simulink model "feedback_control"  (R2020b)
settings: Solver=FixedStepDiscrete  StartTime=0.0  StopTime=inf  FixedStep=step_size  RelTol=1e-3  EnableMultiTasking=on
libraries: arduinolib x1, dspstat3 x1, arduinosensorlib x1
settings Model: DataDictionary=data2.sldd  EnableAccessToBaseWorkspace=off  ModifiedByFormat=The MathWorks Inc.  SILPILModeSetting=veronly  ExtModeTrigDuration=2  Creator=The MathWorks, Inc.  LastModifiedBy=The MathWorks Inc.
settings DataIOCC: SaveFormat=Array  ReturnWorkspaceOutputs=off
settings OptimizationCC: PassReuseOutputArgsAs=Individual arguments  ExpressionDepthLimit=2147483647  ZeroExternalMemoryAtStartup=off  ZeroInternalMemoryAtStartup=off  EfficientFloat2IntCast=on  LifeSpan=1  MaxStackSize=64  EfficientTunableParamExpr=on
settings DebuggingCC: SolverPrmCheckMsg=warning  FcnCallInpInsideContextMsg=warning  UniqueDataStoreMsg=error  AssertControl=DisableAll  AllowSymbolicDim=off  StateNameClashWarn=warning  StrictBusMsg=ErrorOnBusTreatedAsVector  SFUnexpectedBacktrackingDiag=warning  SFNoUnconditionalDefaultTransitionDiag=warning  SFExecutionAtInitializationDiag=none  ArithmeticOperatorsInVariantConditions=warning
settings HardwareCC: ProdBitPerInt=16  ProdBitPerPointer=16  ProdBitPerSizeT=16  ProdBitPerPtrDiffT=16  ProdLargestAtomicFloat=None  ProdWordSize=8  ProdHWDeviceType=Atmel->AVR
settings ModelReferenceCC: PropagateSignalLabelsOutOfModel=off
settings SFSimCC: SimUseLocalCustomCode=off  CustomCodeUndefinedFunction=UseInterfaceOnly
settings RTWCC: Description=Embedded Coder  SystemTargetFile=ert.tlc  HardwareBoard=Arduino Uno  TemplateMakefile=ert_default_tmf  RTWUseLocalCustomCode=off  Toolchain=Arduino AVR  BuildConfiguration=Faster Runs  IncludeHyperlinkInReport=on  GenerateCodeMetricsReport=on
settings CodeAppCC: IgnoreCustomStorageClasses=off  IgnoreTestpoints=on  CustomSymbolStrType=$N$R$M  StateflowObjectComments=on  InternalIdentifier=Classic
settings ERTTargetCC: MultiwordLength=2048  SupportNonFinite=off  SupportContinuousTime=on  SupportVariableSizeSignals=on  ParenthesesLevel=Maximum  ExtModeStaticAllocSize=250  ConvertIfToSwitch=off  SuppressUnreachableDefaultCases=off
settings ConfigComp: CovMetricSettings=dw  CovSaveCumulativeToWorkspaceVar=on  CovSaveSingleToWorkspaceVar=on  CovExternalEMLEnable=off  CovSFcnEnable=off

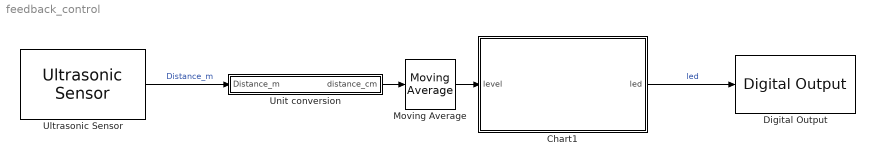
== system feedback_control ==
  Chart1 : Stateflow chart  TreatAsAtomicUnit=on
  Digital Output : arduinolib/Digital Output  pinNumber=13  Direction=output  blockPlatform=arduino
  Moving Average : dspstat3/Moving Average  Method=Sliding window  ForgettingFactorPort=off  SpecifyWindowLength=on  WindowLength=4  ForgettingFactor=0.9  SimulateUsing=Code generation
  Ultrasonic Sensor : arduinosensorlib/Ultrasonic Sensor  NumSignalPins=2  TrigPin=4  EchoPin=5  SignalPin=3  SampleTime_=0.1  blockPlatform=ARDUINO
      settings: SourceProductBaseCode=ARDUINO
  Unit conversion : Subsystem
  wires:
  Chart1/1(led) -> Digital Output/1  "led"
  Ultrasonic Sensor/1 -> Unit conversion/1(Distance_m)  "Distance_m"
  Unit conversion/1(distance_cm) -> Moving Average/1
  Moving Average/1 -> Chart1/1(level)

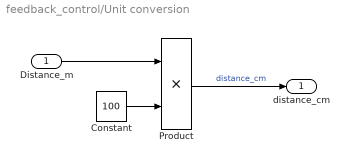
== system feedback_control/Unit conversion ==
  Distance_m : Inport
  Constant : Constant  Value=100
  Product : Product
  distance_cm : Outport
  wires:
  Product/1 -> distance_cm/1  "distance_cm"
  Distance_m/1 -> Product/1
  Constant/1 -> Product/2

== stateflow chart feedback_control/Chart1 ==
  state BLINK_OUTRANGE
    frequency = 0.5;
    state LED_OFF
      entry:
      led = false;
    state LED_ON
      entry:
      led = true;
    (default) -> BLINK_OUTRANGE.LED_ON
    BLINK_OUTRANGE.LED_ON -> BLINK_OUTRANGE.LED_OFF : after(frequency/2, sec)
    BLINK_OUTRANGE.LED_OFF -> BLINK_OUTRANGE.LED_ON : after(frequency/2, sec)
  state BLINK_INRANGE
    frequency = 0.1;
    state LED_OFF
      entry:
      led = false;
    state LED_ON
      entry:
      led = true;
    (default) -> BLINK_INRANGE.LED_ON
    BLINK_INRANGE.LED_OFF -> BLINK_INRANGE.LED_ON : after(frequency - ((level*frequency)/100), sec)
    BLINK_INRANGE.LED_ON -> BLINK_INRANGE.LED_OFF : after((level*frequency)/100, sec)
  state DISCONNECTED_SENSOR
    frequency = 1;
    state LED_OFF
      entry:
      led = false;
    state LED_ON
      entry:
      led = true;
    (default) -> DISCONNECTED_SENSOR.LED_ON
    DISCONNECTED_SENSOR.LED_ON -> DISCONNECTED_SENSOR.LED_OFF : after(frequency/2, sec)
    DISCONNECTED_SENSOR.LED_OFF -> DISCONNECTED_SENSOR.LED_ON : after(frequency/2, sec)
  BLINK_OUTRANGE -> BLINK_INRANGE [order 1] : [level >=10 && level <=100]
  BLINK_INRANGE -> BLINK_OUTRANGE : [level < 10 || level >100]
  (default) -> DISCONNECTED_SENSOR
  (junction 156) -> BLINK_OUTRANGE
  BLINK_OUTRANGE -> (junction 136) [order 2] : [level == 0]
  (junction 174) -> BLINK_INRANGE
  (junction 136) -> DISCONNECTED_SENSOR
  DISCONNECTED_SENSOR -> (junction 174) [order 2] : [level >=10 && level <=100]
  DISCONNECTED_SENSOR -> (junction 156) [order 1] : [level ~= 0 && ( level < 10 || level > 100 )]
  data: led output boolean; frequency local single; level input double
